simulink model "wk4sim_linear"  (R2021b)
settings: Solver=VariableStepAuto  StartTime=0.0  StopTime=10.0  RelTol=1e-3
undefined symbols (not defined in the file): A, B, C, D, Force, x0
settings Model: Creator=Cyril  LastModifiedBy=Cyril

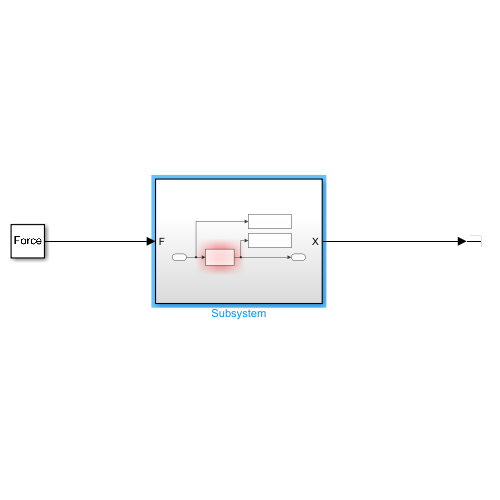
[thumbnail: Simulink's stored preview of the top-level diagram]
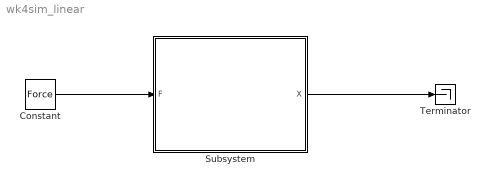
== system wk4sim_linear ==
  Constant : Constant  Value=Force
  Subsystem : Subsystem
  Terminator : Terminator
  wires:
  Constant/1 -> Subsystem/1(F)
  Subsystem/1(X) -> Terminator/1

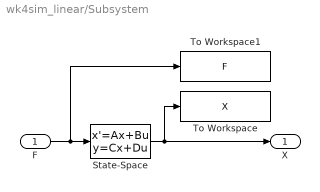
== system wk4sim_linear/Subsystem ==
  F : Inport
  State-Space : StateSpace  A=A  B=B  C=C  D=D  InitialCondition=x0
  To Workspace : ToWorkspace  VariableName=X  SampleTime=-1
  To Workspace1 : ToWorkspace  VariableName=F  SampleTime=-1
  X : Outport
  wires:
  F/1 -> To Workspace1/1, State-Space/1
  State-Space/1 -> To Workspace/1, X/1
